simulink model "part_3_sim_w_car"  (R2018b)
settings: Solver=VariableStepAuto  StartTime=0.0  StopTime=t_f  MaxStep=.001  RelTol=1e-3  EnableMultiTasking=on
values from neighbouring files (symbols this model uses):
  alpha_final = 3*pi/180    (= 0.0523598775598)    [Part_3.m]
  alpha_initial = 0    [Part_3.m]
  alpha_step_time = 15    [Part_3.m]
  b = 62    [Part_3.m]
  bar_i_a = double(Y.a(2))    [Part_3.m]
  bar_i_f = double(Y.f(2))    [Part_3.m]
  bar_v = double(Y.v(2))    [Part_3.m]
  bar_vel = 26.8224    [Part_3.m]
  D = 0.48    [Part_3.m]
  Delta = 9.73    [Part_3.m]
  g = 9.81    [Part_3.m]
  G1 = tf(zpk([-0.065],[-0.013],[41]))    [Part_3.m]
  k_b = 1.4e-4    (= 0.00014)    [Part_3.m]
  l = 0.5    [Part_3.m]
  La = 0.005    [Part_3.m]
  Lf = 0.3    [Part_3.m]
  m = 2110    [Part_3.m]
  N = 126    [Part_3.m]
  r = 1/6    (= 0.166666666667)    [Part_3.m]
  Ra = 0.07    [Part_3.m]
  Rf = 6.5    [Part_3.m]
  v_final = 31.2928    [Part_3.m]
  v_initial = 26.8224    [Part_3.m]
  v_step_time = 1    [Part_3.m]
libraries: simulink x13
settings Model: Creator=hoelzle.1  LastModifiedBy=Nick Carcione
settings OptimizationCC: LifeSpan=inf
settings DebuggingCC: SFUnexpectedBacktrackingDiag=warning  SFNoUnconditionalDefaultTransitionDiag=warning
settings SFSimCC: SimUseLocalCustomCode=off
settings RTWCC: RTWUseLocalCustomCode=off
settings CodeAppCC: StateflowObjectComments=on
settings GRTTargetCC: TargetLangStandard=C89/C90 (ANSI)  GeneratePreprocessorConditionals=Disable all
settings ConfigComp: CovMetricSettings=dw  CovHtmlReporting=on  CovSaveCumulativeToWorkspaceVar=on  CovSaveSingleToWorkspaceVar=on  CovExternalEMLEnable=off

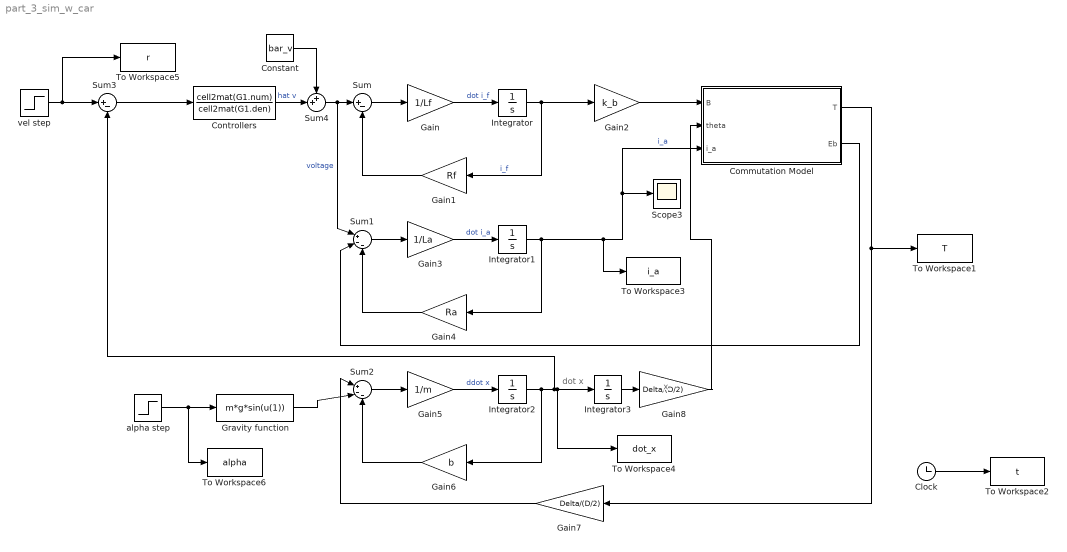
== system part_3_sim_w_car ==
  note: x
  note: dot x
  Clock : Clock
  Commutation Model : Subsystem
  Constant : Constant  Value=bar_v
  Controllers : TransferFcn  Numerator=cell2mat(G1.num)  Denominator=cell2mat(G1.den)
  Gain : Gain  Gain=1/Lf
  Gain1 : Gain  Gain=Rf
  Gain2 : Gain  Gain=k_b
  Gain3 : Gain  Gain=1/La
  Gain4 : Gain  Gain=Ra
  Gain5 : Gain  Gain=1/m
  Gain6 : Gain  Gain=b
  Gain7 : Gain  Gain=Delta/(D/2)
  Gain8 : Gain  Gain=Delta/(D/2)
  Gravity function : Fcn  Expr=m*g*sin(u(1))
  Integrator : Integrator  InitialCondition=bar_i_f
  Integrator1 : Integrator  InitialCondition=bar_i_a
  Integrator2 : Integrator  InitialCondition=bar_vel
  Integrator3 : Integrator
  Scope3 : Scope
  Sum : Sum  Inputs=|+-
  Sum1 : Sum  Inputs=|+--
  Sum2 : Sum  Inputs=|+--
  Sum3 : Sum  Inputs=|+-
  Sum4 : Sum  Inputs=++|
  To Workspace1 : ToWorkspace  VariableName=T  SampleTime=-1
  To Workspace2 : ToWorkspace  VariableName=t  SampleTime=-1
  To Workspace3 : ToWorkspace  VariableName=i_a  SampleTime=-1
  To Workspace4 : ToWorkspace  VariableName=dot_x  SampleTime=-1
  To Workspace5 : ToWorkspace  VariableName=r  SampleTime=-1
  To Workspace6 : ToWorkspace  VariableName=alpha  SampleTime=-1
  alpha step : Step  Time=alpha_step_time  Before=alpha_initial  After=alpha_final  SampleTime=0
  "vel step " : Step  Time=v_step_time  Before=v_initial  After=v_final  SampleTime=0
  wires:
  Clock/1 -> To Workspace2/1
  Sum/1 -> Gain/1
  Gain/1 -> Integrator/1  "dot i_f"
  Integrator/1 -> Gain2/1, Gain1/1  "i_f"
  Gain2/1 -> Commutation Model/1(B)
  Sum1/1 -> Gain3/1
  Gain3/1 -> Integrator1/1  "dot i_a"
  Integrator1/1 -> To Workspace3/1, Scope3/1, Commutation Model/3(i_a), Gain4/1  "i_a"
  Gain4/1 -> Sum1/3
  Commutation Model/2(Eb) -> Sum1/2
  Sum2/1 -> Gain5/1
  Gain5/1 -> Integrator2/1  "ddot x"
  Commutation Model/1(T) -> To Workspace1/1, Gain7/1
  Gain7/1 -> Sum2/1
  Integrator3/1 -> Gain8/1
  Gain8/1 -> Commutation Model/2(theta)
  Gain6/1 -> Sum2/3
  Gravity function/1 -> Sum2/2
  alpha step/1 -> To Workspace6/1, Gravity function/1
  "vel step "/1 -> To Workspace5/1, Sum3/1
  Sum3/1 -> Controllers/1
  Integrator2/1 -> To Workspace4/1, Integrator3/1, Sum3/2, Gain6/1
  Gain1/1 -> Sum/2
  Controllers/1 -> Sum4/2  "hat v"
  Sum4/1 -> Sum1/1, Sum/1  "voltage"
  Constant/1 -> Sum4/1

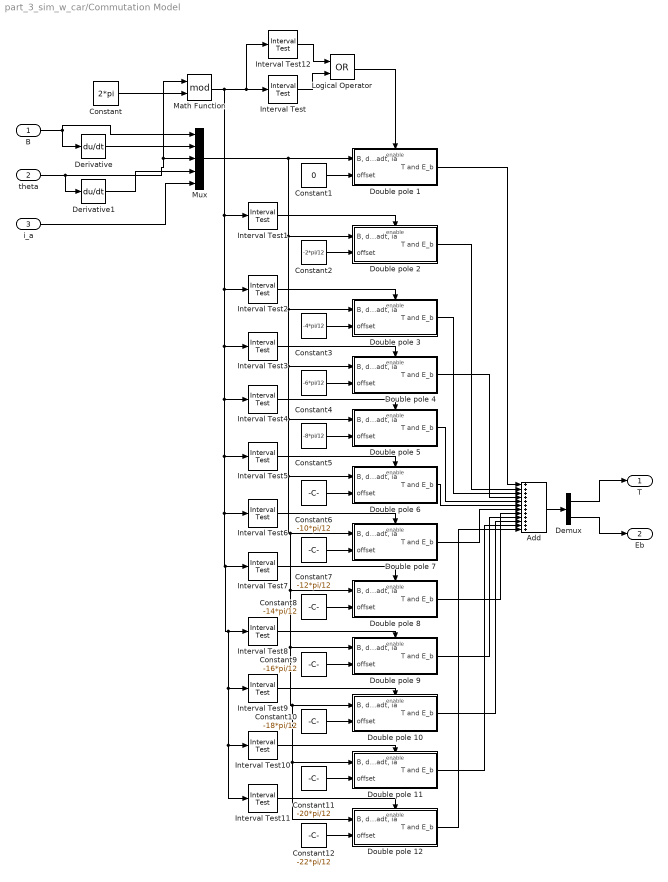
== system part_3_sim_w_car/Commutation Model ==
  B : Inport
  theta : Inport  Port=2
  i_a : Inport  Port=3
  Add : Sum  Inputs=++++++++++++
  Constant : Constant  Value=2*pi
  Constant1 : Constant  Value=0
  Constant10 : Constant  Value=-18*pi/12
  Constant11 : Constant  Value=-20*pi/12
  Constant12 : Constant  Value=-22*pi/12
  Constant2 : Constant  Value=-2*pi/12
  Constant3 : Constant  Value=-4*pi/12
  Constant4 : Constant  Value=-6*pi/12
  Constant5 : Constant  Value=-8*pi/12
  Constant6 : Constant  Value=-10*pi/12
  Constant7 : Constant  Value=-12*pi/12
  Constant8 : Constant  Value=-14*pi/12
  Constant9 : Constant  Value=-16*pi/12
  Demux : Demux  Outputs=2
  Derivative : Derivative
  Derivative1 : Derivative
  Double pole 1 : Subsystem
  Double pole 10 : Subsystem
  Double pole 11 : Subsystem
  Double pole 12 : Subsystem
  Double pole 2 : Subsystem
  Double pole 3 : Subsystem
  Double pole 4 : Subsystem
  Double pole 5 : Subsystem
  Double pole 6 : Subsystem
  Double pole 7 : Subsystem
  Double pole 8 : Subsystem
  Double pole 9 : Subsystem
  Interval Test : simulink/Logic and Bit Operations/Interval Test  IntervalClosedRight=off  uplimit=pi/12  IntervalClosedLeft=on  lowlimit=0  OutDataTypeStr=boolean
  Interval Test1 : simulink/Logic and Bit Operations/Interval Test  IntervalClosedRight=off  uplimit=3*pi/12  IntervalClosedLeft=on  lowlimit=pi/12  OutDataTypeStr=boolean
  Interval Test10 : simulink/Logic and Bit Operations/Interval Test  IntervalClosedRight=off  uplimit=21*pi/12  IntervalClosedLeft=on  lowlimit=19*pi/12  OutDataTypeStr=boolean
  Interval Test11 : simulink/Logic and Bit Operations/Interval Test  IntervalClosedRight=off  uplimit=23*pi/12  IntervalClosedLeft=on  lowlimit=21*pi/12  OutDataTypeStr=boolean
  Interval Test12 : simulink/Logic and Bit Operations/Interval Test  IntervalClosedRight=on  uplimit=24*pi/12  IntervalClosedLeft=on  lowlimit=23*pi/12  OutDataTypeStr=boolean
  Interval Test2 : simulink/Logic and Bit Operations/Interval Test  IntervalClosedRight=off  uplimit=5*pi/12  IntervalClosedLeft=on  lowlimit=3*pi/12  OutDataTypeStr=boolean
  Interval Test3 : simulink/Logic and Bit Operations/Interval Test  IntervalClosedRight=off  uplimit=7*pi/12  IntervalClosedLeft=on  lowlimit=5*pi/12  OutDataTypeStr=boolean
  Interval Test4 : simulink/Logic and Bit Operations/Interval Test  IntervalClosedRight=off  uplimit=9*pi/12  IntervalClosedLeft=on  lowlimit=7*pi/12  OutDataTypeStr=boolean
  Interval Test5 : simulink/Logic and Bit Operations/Interval Test  IntervalClosedRight=off  uplimit=11*pi/12  IntervalClosedLeft=on  lowlimit=9*pi/12  OutDataTypeStr=boolean
  Interval Test6 : simulink/Logic and Bit Operations/Interval Test  IntervalClosedRight=off  uplimit=13*pi/12  IntervalClosedLeft=on  lowlimit=11*pi/12  OutDataTypeStr=boolean
  Interval Test7 : simulink/Logic and Bit Operations/Interval Test  IntervalClosedRight=off  uplimit=15*pi/12  IntervalClosedLeft=on  lowlimit=13*pi/12  OutDataTypeStr=boolean
  Interval Test8 : simulink/Logic and Bit Operations/Interval Test  IntervalClosedRight=off  uplimit=17*pi/12  IntervalClosedLeft=on  lowlimit=15*pi/12  OutDataTypeStr=boolean
  Interval Test9 : simulink/Logic and Bit Operations/Interval Test  IntervalClosedRight=off  uplimit=19*pi/12  IntervalClosedLeft=on  lowlimit=17*pi/12  OutDataTypeStr=boolean
  Logical Operator : Logic  Operator=OR  AllPortsSameDT=off  OutDataTypeStr=boolean
  Math Function : Math  Operator=mod  SaturateOnIntegerOverflow=on
  Mux : Mux  Inputs=5
  T : Outport
  Eb : Outport  Port=2
  wires:
  B/1 -> Derivative/1, Mux/1
  theta/1 -> Derivative1/1, Mux/3, Math Function/1
  Double pole 1/1(T and E_b) -> Add/1
  Constant/1 -> Math Function/2
  Math Function/1 -> Interval Test11/1, Interval Test10/1, Interval Test9/1, Interval Test8/1, Interval Test7/1, Interval Test6/1, Interval Test5/1, Interval Test4/1, Interval Test3/1, Interval Test2/1, Interval Test1/1, Interval Test12/1, Interval Test/1
  Logical Operator/1 -> Double pole 1/Enable
  Interval Test/1 -> Logical Operator/2
  Interval Test12/1 -> Logical Operator/1
  Derivative/1 -> Mux/2
  Derivative1/1 -> Mux/4
  i_a/1 -> Mux/5
  Mux/1 -> Double pole 12/1("B, dBdt, theta, dthetadt, ia"), Double pole 11/1("B, dBdt, theta, dthetadt, ia"), Double pole 10/1("B, dBdt, theta, dthetadt, ia"), Double pole 9/1("B, dBdt, theta, dthetadt, ia"), Double pole 8/1("B, dBdt, theta, dthetadt, ia"), Double pole 7/1("B, dBdt, theta, dthetadt, ia"), Double pole 6/1("B, dBdt, theta, dthetadt, ia"), Double pole 5/1("B, dBdt, theta, dthetadt, ia"), Double pole 4/1("B, dBdt, theta, dthetadt, ia"), Double pole 3/1("B, dBdt, theta, dthetadt, ia"), Double pole 2/1("B, dBdt, theta, dthetadt, ia"), Double pole 1/1("B, dBdt, theta, dthetadt, ia")
  Constant1/1 -> Double pole 1/2(offset)
  Constant2/1 -> Double pole 2/2(offset)
  Constant3/1 -> Double pole 3/2(offset)
  Constant4/1 -> Double pole 4/2(offset)
  Constant5/1 -> Double pole 5/2(offset)
  Constant6/1 -> Double pole 6/2(offset)
  Constant7/1 -> Double pole 7/2(offset)
  Constant8/1 -> Double pole 8/2(offset)
  Constant9/1 -> Double pole 9/2(offset)
  Constant10/1 -> Double pole 10/2(offset)
  Constant11/1 -> Double pole 11/2(offset)
  Constant12/1 -> Double pole 12/2(offset)
  Interval Test1/1 -> Double pole 2/Enable
  Interval Test2/1 -> Double pole 3/Enable
  Interval Test3/1 -> Double pole 4/Enable
  Interval Test4/1 -> Double pole 5/Enable
  Interval Test5/1 -> Double pole 6/Enable
  Interval Test6/1 -> Double pole 7/Enable
  Interval Test7/1 -> Double pole 8/Enable
  Interval Test8/1 -> Double pole 9/Enable
  Interval Test9/1 -> Double pole 10/Enable
  Interval Test10/1 -> Double pole 11/Enable
  Interval Test11/1 -> Double pole 12/Enable
  Add/1 -> Demux/1
  Demux/1 -> T/1
  Demux/2 -> Eb/1
  Double pole 2/1(T and E_b) -> Add/2
  Double pole 3/1(T and E_b) -> Add/3
  Double pole 4/1(T and E_b) -> Add/4
  Double pole 5/1(T and E_b) -> Add/5
  Double pole 6/1(T and E_b) -> Add/6
  Double pole 7/1(T and E_b) -> Add/7
  Double pole 8/1(T and E_b) -> Add/8
  Double pole 9/1(T and E_b) -> Add/9
  Double pole 10/1(T and E_b) -> Add/10
  Double pole 11/1(T and E_b) -> Add/11
  Double pole 12/1(T and E_b) -> Add/12

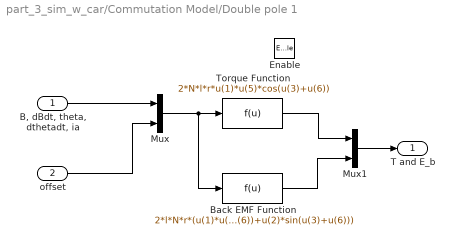
== system part_3_sim_w_car/Commutation Model/Double pole 1 ==
  "B, dBdt, theta, dthetadt, ia" : Inport
  offset : Inport  Port=2
  Enable : EnablePort
  Back EMF Function : Fcn  Expr=2*l*N*r*(u(1)*u(4)*cos(u(3)+u(6))+u(2)*sin(u(3)+u(6)))
  Mux : Mux  Inputs=2
  Mux1 : Mux  Inputs=2
  Torque Function : Fcn  Expr=2*N*l*r*u(1)*u(5)*cos(u(3)+u(6))
  T and E_b : Outport  OutputWhenDisabled=reset  InitialOutput=[0]
  wires:
  "B, dBdt, theta, dthetadt, ia"/1 -> Mux/1
  offset/1 -> Mux/2
  Mux/1 -> Back EMF Function/1, Torque Function/1
  Torque Function/1 -> Mux1/1
  Back EMF Function/1 -> Mux1/2
  Mux1/1 -> T and E_b/1

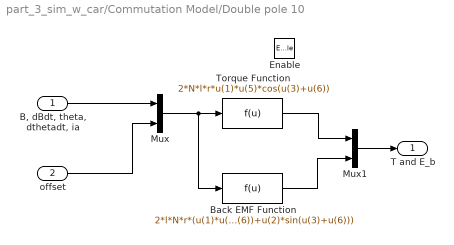
== system part_3_sim_w_car/Commutation Model/Double pole 10 ==
  "B, dBdt, theta, dthetadt, ia" : Inport
  offset : Inport  Port=2
  Enable : EnablePort
  Back EMF Function : Fcn  Expr=2*l*N*r*(u(1)*u(4)*cos(u(3)+u(6))+u(2)*sin(u(3)+u(6)))
  Mux : Mux  Inputs=2
  Mux1 : Mux  Inputs=2
  Torque Function : Fcn  Expr=2*N*l*r*u(1)*u(5)*cos(u(3)+u(6))
  T and E_b : Outport  OutputWhenDisabled=reset  InitialOutput=[0]
  wires:
  "B, dBdt, theta, dthetadt, ia"/1 -> Mux/1
  offset/1 -> Mux/2
  Mux/1 -> Back EMF Function/1, Torque Function/1
  Torque Function/1 -> Mux1/1
  Back EMF Function/1 -> Mux1/2
  Mux1/1 -> T and E_b/1

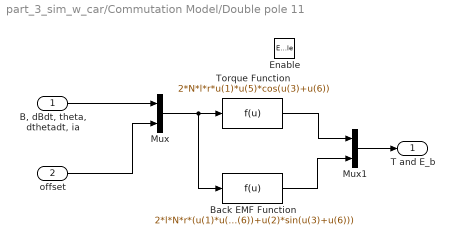
== system part_3_sim_w_car/Commutation Model/Double pole 11 ==
  "B, dBdt, theta, dthetadt, ia" : Inport
  offset : Inport  Port=2
  Enable : EnablePort
  Back EMF Function : Fcn  Expr=2*l*N*r*(u(1)*u(4)*cos(u(3)+u(6))+u(2)*sin(u(3)+u(6)))
  Mux : Mux  Inputs=2
  Mux1 : Mux  Inputs=2
  Torque Function : Fcn  Expr=2*N*l*r*u(1)*u(5)*cos(u(3)+u(6))
  T and E_b : Outport  OutputWhenDisabled=reset  InitialOutput=[0]
  wires:
  "B, dBdt, theta, dthetadt, ia"/1 -> Mux/1
  offset/1 -> Mux/2
  Mux/1 -> Back EMF Function/1, Torque Function/1
  Torque Function/1 -> Mux1/1
  Back EMF Function/1 -> Mux1/2
  Mux1/1 -> T and E_b/1

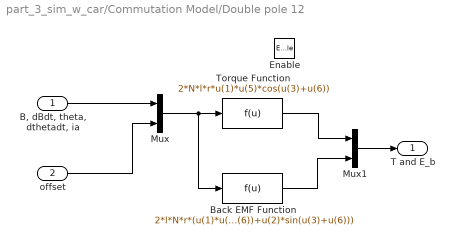
== system part_3_sim_w_car/Commutation Model/Double pole 12 ==
  "B, dBdt, theta, dthetadt, ia" : Inport
  offset : Inport  Port=2
  Enable : EnablePort
  Back EMF Function : Fcn  Expr=2*l*N*r*(u(1)*u(4)*cos(u(3)+u(6))+u(2)*sin(u(3)+u(6)))
  Mux : Mux  Inputs=2
  Mux1 : Mux  Inputs=2
  Torque Function : Fcn  Expr=2*N*l*r*u(1)*u(5)*cos(u(3)+u(6))
  T and E_b : Outport  OutputWhenDisabled=reset  InitialOutput=[0]
  wires:
  "B, dBdt, theta, dthetadt, ia"/1 -> Mux/1
  offset/1 -> Mux/2
  Mux/1 -> Back EMF Function/1, Torque Function/1
  Torque Function/1 -> Mux1/1
  Back EMF Function/1 -> Mux1/2
  Mux1/1 -> T and E_b/1

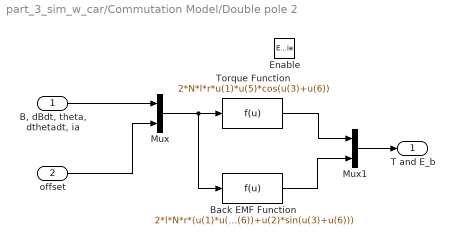
== system part_3_sim_w_car/Commutation Model/Double pole 2 ==
  "B, dBdt, theta, dthetadt, ia" : Inport
  offset : Inport  Port=2
  Enable : EnablePort
  Back EMF Function : Fcn  Expr=2*l*N*r*(u(1)*u(4)*cos(u(3)+u(6))+u(2)*sin(u(3)+u(6)))
  Mux : Mux  Inputs=2
  Mux1 : Mux  Inputs=2
  Torque Function : Fcn  Expr=2*N*l*r*u(1)*u(5)*cos(u(3)+u(6))
  T and E_b : Outport  OutputWhenDisabled=reset  InitialOutput=[0]
  wires:
  "B, dBdt, theta, dthetadt, ia"/1 -> Mux/1
  offset/1 -> Mux/2
  Mux/1 -> Back EMF Function/1, Torque Function/1
  Torque Function/1 -> Mux1/1
  Back EMF Function/1 -> Mux1/2
  Mux1/1 -> T and E_b/1

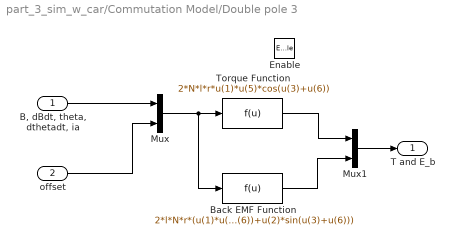
== system part_3_sim_w_car/Commutation Model/Double pole 3 ==
  "B, dBdt, theta, dthetadt, ia" : Inport
  offset : Inport  Port=2
  Enable : EnablePort
  Back EMF Function : Fcn  Expr=2*l*N*r*(u(1)*u(4)*cos(u(3)+u(6))+u(2)*sin(u(3)+u(6)))
  Mux : Mux  Inputs=2
  Mux1 : Mux  Inputs=2
  Torque Function : Fcn  Expr=2*N*l*r*u(1)*u(5)*cos(u(3)+u(6))
  T and E_b : Outport  OutputWhenDisabled=reset  InitialOutput=[0]
  wires:
  "B, dBdt, theta, dthetadt, ia"/1 -> Mux/1
  offset/1 -> Mux/2
  Mux/1 -> Back EMF Function/1, Torque Function/1
  Torque Function/1 -> Mux1/1
  Back EMF Function/1 -> Mux1/2
  Mux1/1 -> T and E_b/1

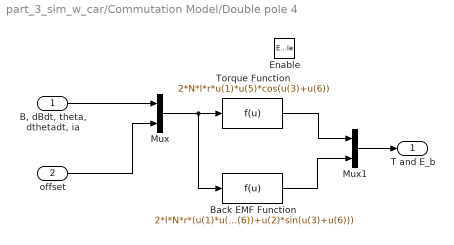
== system part_3_sim_w_car/Commutation Model/Double pole 4 ==
  "B, dBdt, theta, dthetadt, ia" : Inport
  offset : Inport  Port=2
  Enable : EnablePort
  Back EMF Function : Fcn  Expr=2*l*N*r*(u(1)*u(4)*cos(u(3)+u(6))+u(2)*sin(u(3)+u(6)))
  Mux : Mux  Inputs=2
  Mux1 : Mux  Inputs=2
  Torque Function : Fcn  Expr=2*N*l*r*u(1)*u(5)*cos(u(3)+u(6))
  T and E_b : Outport  OutputWhenDisabled=reset  InitialOutput=[0]
  wires:
  "B, dBdt, theta, dthetadt, ia"/1 -> Mux/1
  offset/1 -> Mux/2
  Mux/1 -> Back EMF Function/1, Torque Function/1
  Torque Function/1 -> Mux1/1
  Back EMF Function/1 -> Mux1/2
  Mux1/1 -> T and E_b/1

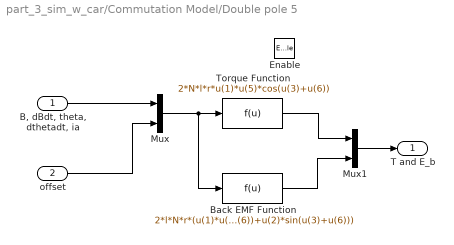
== system part_3_sim_w_car/Commutation Model/Double pole 5 ==
  "B, dBdt, theta, dthetadt, ia" : Inport
  offset : Inport  Port=2
  Enable : EnablePort
  Back EMF Function : Fcn  Expr=2*l*N*r*(u(1)*u(4)*cos(u(3)+u(6))+u(2)*sin(u(3)+u(6)))
  Mux : Mux  Inputs=2
  Mux1 : Mux  Inputs=2
  Torque Function : Fcn  Expr=2*N*l*r*u(1)*u(5)*cos(u(3)+u(6))
  T and E_b : Outport  OutputWhenDisabled=reset  InitialOutput=[0]
  wires:
  "B, dBdt, theta, dthetadt, ia"/1 -> Mux/1
  offset/1 -> Mux/2
  Mux/1 -> Back EMF Function/1, Torque Function/1
  Torque Function/1 -> Mux1/1
  Back EMF Function/1 -> Mux1/2
  Mux1/1 -> T and E_b/1

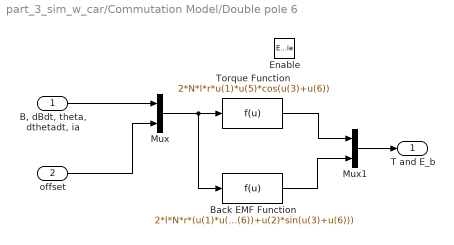
== system part_3_sim_w_car/Commutation Model/Double pole 6 ==
  "B, dBdt, theta, dthetadt, ia" : Inport
  offset : Inport  Port=2
  Enable : EnablePort
  Back EMF Function : Fcn  Expr=2*l*N*r*(u(1)*u(4)*cos(u(3)+u(6))+u(2)*sin(u(3)+u(6)))
  Mux : Mux  Inputs=2
  Mux1 : Mux  Inputs=2
  Torque Function : Fcn  Expr=2*N*l*r*u(1)*u(5)*cos(u(3)+u(6))
  T and E_b : Outport  OutputWhenDisabled=reset  InitialOutput=[0]
  wires:
  "B, dBdt, theta, dthetadt, ia"/1 -> Mux/1
  offset/1 -> Mux/2
  Mux/1 -> Back EMF Function/1, Torque Function/1
  Torque Function/1 -> Mux1/1
  Back EMF Function/1 -> Mux1/2
  Mux1/1 -> T and E_b/1

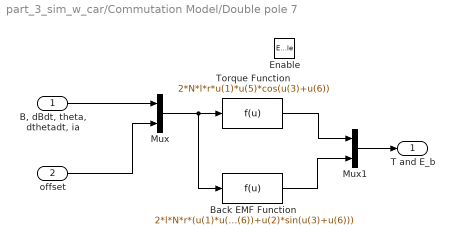
== system part_3_sim_w_car/Commutation Model/Double pole 7 ==
  "B, dBdt, theta, dthetadt, ia" : Inport
  offset : Inport  Port=2
  Enable : EnablePort
  Back EMF Function : Fcn  Expr=2*l*N*r*(u(1)*u(4)*cos(u(3)+u(6))+u(2)*sin(u(3)+u(6)))
  Mux : Mux  Inputs=2
  Mux1 : Mux  Inputs=2
  Torque Function : Fcn  Expr=2*N*l*r*u(1)*u(5)*cos(u(3)+u(6))
  T and E_b : Outport  OutputWhenDisabled=reset  InitialOutput=[0]
  wires:
  "B, dBdt, theta, dthetadt, ia"/1 -> Mux/1
  offset/1 -> Mux/2
  Mux/1 -> Back EMF Function/1, Torque Function/1
  Torque Function/1 -> Mux1/1
  Back EMF Function/1 -> Mux1/2
  Mux1/1 -> T and E_b/1

== system part_3_sim_w_car/Commutation Model/Double pole 8 ==
  "B, dBdt, theta, dthetadt, ia" : Inport
  offset : Inport  Port=2
  Enable : EnablePort
  Back EMF Function : Fcn  Expr=2*l*N*r*(u(1)*u(4)*cos(u(3)+u(6))+u(2)*sin(u(3)+u(6)))
  Mux : Mux  Inputs=2
  Mux1 : Mux  Inputs=2
  Torque Function : Fcn  Expr=2*N*l*r*u(1)*u(5)*cos(u(3)+u(6))
  T and E_b : Outport  OutputWhenDisabled=reset  InitialOutput=[0]
  wires:
  "B, dBdt, theta, dthetadt, ia"/1 -> Mux/1
  offset/1 -> Mux/2
  Mux/1 -> Back EMF Function/1, Torque Function/1
  Torque Function/1 -> Mux1/1
  Back EMF Function/1 -> Mux1/2
  Mux1/1 -> T and E_b/1

== system part_3_sim_w_car/Commutation Model/Double pole 9 ==
  "B, dBdt, theta, dthetadt, ia" : Inport
  offset : Inport  Port=2
  Enable : EnablePort
  Back EMF Function : Fcn  Expr=2*l*N*r*(u(1)*u(4)*cos(u(3)+u(6))+u(2)*sin(u(3)+u(6)))
  Mux : Mux  Inputs=2
  Mux1 : Mux  Inputs=2
  Torque Function : Fcn  Expr=2*N*l*r*u(1)*u(5)*cos(u(3)+u(6))
  T and E_b : Outport  OutputWhenDisabled=reset  InitialOutput=[0]
  wires:
  "B, dBdt, theta, dthetadt, ia"/1 -> Mux/1
  offset/1 -> Mux/2
  Mux/1 -> Back EMF Function/1, Torque Function/1
  Torque Function/1 -> Mux1/1
  Back EMF Function/1 -> Mux1/2
  Mux1/1 -> T and E_b/1
